simulink model "OilSim"  (R2025b)
settings: Solver=VariableStepAuto  StartTime=0.0  StopTime=500  RelTol=1e-3
libraries: cstblocks x1, mpclib x1
settings Model: Creator=shamanth  LastModifiedBy=shamanth

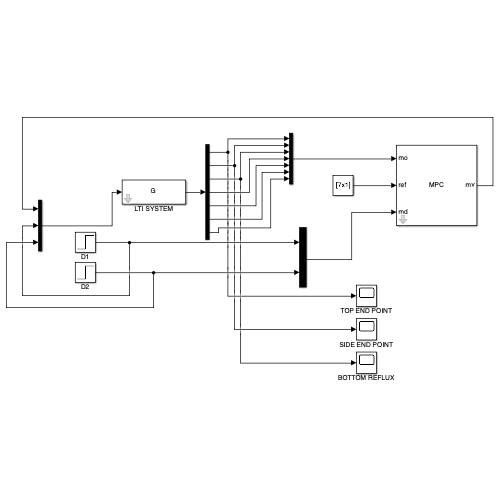
[thumbnail: Simulink's stored preview of the top-level diagram]
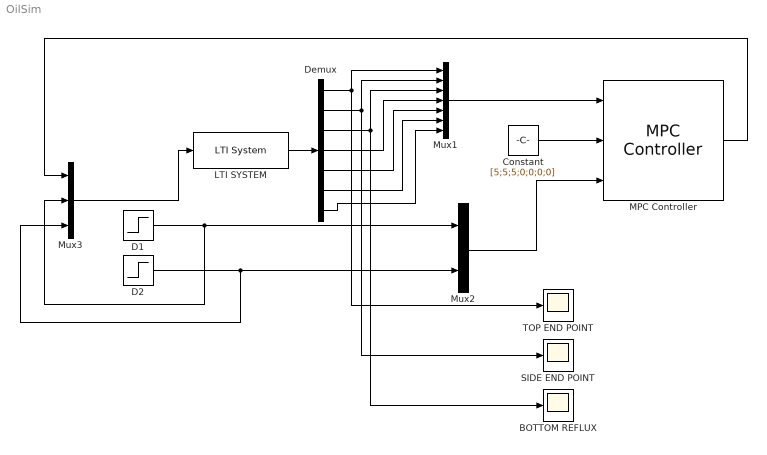
== system OilSim ==
  BOTTOM REFLUX : Scope
      settings: ActiveDisplayYMinimum=-0.63427018997125562  ActiveDisplayYMaximum=5.7084317097413013  DataLoggingVariableName=ScopeData2
  Constant : Constant  Value=[5;5;5;0;0;0;0]
  D1 : Step  After=0.5  SampleTime=0
  D2 : Step  After=0.5  SampleTime=0
  Demux : Demux  Outputs=7
  LTI SYSTEM : cstblocks/LTI System  sys=G  IC=[]  PadeOrder=0
  MPC Controller : mpclib/MPC Controller  SCDEnableBlockLinearizationSpecification=on  mpcobj=mpcobj  is_multiple=0  enable_value=0  return_u0=off  updateMPCinCallerWorkspace=on  md_inport=on  mv_inport=off  uref_inport=off  return_cost=off  return_mvseq=off  return_qpstatus=off  return_xseq=off  return_state=off  return_ovseq=off  state_inport=off  umin_inport=off  umax_inport=off  ymin_inport=off  ymax_inport=off  cc_inport=off  ywt_inport=off  uwt_inport=off  duwt_inport=off  rhoeps_inport=off  pm_inport=off  MaximumP=10  HorizonChoice=FixedHorizon  n_ts=2  n_p=90  n_mv=3  n_md=2  n_ud=0  n_mo=7  n_uo=0  BlockDataType=double  SampleTimeInherited=off  switch_inport=off
  Mux1 : Mux  Inputs=7
  Mux2 : Mux  Inputs=2
  Mux3 : Mux  Inputs=3
  SIDE END POINT : Scope
      settings: ActiveDisplayYMinimum=-0.65864113939978275  ActiveDisplayYMaximum=5.9277702545980455
  TOP END POINT : Scope
      settings: ActiveDisplayYMinimum=-0.69777217144836212  ActiveDisplayYMaximum=6.27994954303526
  wires:
  LTI SYSTEM/1 -> Demux/1
  Demux/1 -> TOP END POINT/1, Mux1/1
  Demux/2 -> SIDE END POINT/1, Mux1/2
  Mux1/1 -> MPC Controller/1
  Constant/1 -> MPC Controller/2
  D1/1 -> Mux3/2, Mux2/1
  D2/1 -> Mux3/3, Mux2/2
  Mux2/1 -> MPC Controller/3
  Demux/3 -> BOTTOM REFLUX/1, Mux1/3
  Demux/4 -> Mux1/4
  Demux/5 -> Mux1/5
  Demux/6 -> Mux1/6
  Demux/7 -> Mux1/7
  MPC Controller/1 -> Mux3/1
  Mux3/1 -> LTI SYSTEM/1
